simulink model "Example_IOBlock_Library_CAN"  (Simulink 10.3)
settings: Solver=FixedStepDiscrete  StartTime=0.0  StopTime=10.0  FixedStep=0.01  RelTol=1e-3
libraries: IOBlock_Library_TTC580 x18, simulink x2
settings Model: Creator=hokka  LastModifiedBy=knovakovic  MultithreadedSim=on
settings Model: SuppressorTable=|
  | <?xml version="1.0" encoding="UTF-8" standalone="yes" ?>
  | <!DOCTYPE boost_serialization>
  | <boost_serialization signature="serialization::archive" version="17">
  | <DiagnosticSuppressor class_id="0" tracking_level="0" version="7">
  | 	<Table class_id="1" tracking_level="0" version="0">
  | 		<count>4</count>
  | 		<bucket_count>8</bucket_count>
  | 		<item_version>0</item_version>
  | 		<item class_id="2" tracking_level="0" version="0">
  | 			<first class_id="3" tracking_level="0" version="7">
  | 				<Source class_id="4" tracking_level="0" version="0">
  | 					<count>1</count>
  | 					<item_version>0</item_version>
  | 					<item>57:2245</item>
  | 				</Source>
  | 			</first>
  | 			<second class_id="5" tracking_level="0" version="7">
  | 				<SuppressedData class_id="6" tracking_level="0" version="0">
  | 					<count>2</count>
  | 					<bucket_count>8</bucket_count>
  | 					<item_version>0</item_version>
  | 					<item class_id="7" tracking_level="0" version="0">
  | 						<first class_id="8" tracking_level="0" version="7">
  | 							<ID>SimulinkFixedPoint:util:Overflowoccurred</ID>
  | 							<Cause>
  | 								<Source>
  | 									<count>0</count>
  | 									<item_version>0</item_version>
  | 								</Source>
  | 							</Cause>
  | 						</first>
  | 						<second class_id="9" tracking_level="0" version="7">
  | 							<Comment></Comment>
  | 							<User></User>
  | 							<LastModified class_id="10" tracking_level="0" version="0">
  | 								<ptime_date class_id="11" tracking_level="0" version="0">
  | 									<date>20160608</date>
  | 								</ptime_date>
  | 								<ptime_time_duration class_id="12" tracking_level="0" version="1">
  | 									<is_special>0</is_special>
  | 									<time_duration_hours>15</time_duration_hours>
  | 									<time_duration_minutes>23</time_duration_minutes>
  | 									<time_duration_seconds>17</time_duration_seconds>
  | 									<time_duration_fractional_seconds>0</time_duration_fractional_seconds>
  | 								</ptime_time_duration>
  | 							</LastModified>
  | 							<SuppressionType>1</SuppressionType>
  | 						</second>
  | 					</item>
  | 					<item>
  | 						<first>
  | 							<ID>Simulink:DataType:WarningOverFlowDetected</ID>
  | 							<Cause>
  | 								<Source>
  | 									<count>0</count>
  | 									<item_version>0</item_version>
  | 								</Source>
  | 							</Cause>
  | 						</first>
  | 						<second>
  | 							<Comment></Comment>
  | 							<User></User>
  | 							<LastModified>
  | 								<ptime_date>
  | 									<date>20160608</date>
  | 								</ptime_date>
  | 								<ptime_time_duration>
  | 									<is_special>0</is_special>
  | 									<time_duration_hours>15</time_duration_hours>
  | 									<time_duration_minutes>23</time_duration_minutes>
  | 									<time_duration_seconds>17</time_duration_seconds>
  | 									<time_duration_fractional_seconds>0</time_duration_fractional_seconds>
  | 								</ptime_time_duration>
  | 							</LastModified>
  | 							<SuppressionType>1</SuppressionType>
  | 						</second>
  | 					</item>
  | 				</SuppressedData>
  | 			</second>
  | 		</item>
  | 		<item>
  | 			<first>
  | 				<Source>
  | 					<count>1</count>
  | 					<item_version>0</item_version>
  | 					<item>56:2245</item>
  | 				</Source>
  | 			</first>
  | 			<second>
  | 				<SuppressedData>
  | 					<count>2</count>
  | 					<bucket_count>8</bucket_count>
  | 					<item_version>0</item_version>
  | 					<item>
  | 						<first>
  | 							<ID>SimulinkFixedPoint:util:Overflowoccurred</ID>
  | 							<Cause>
  | 								<Source>
  | 									<count>0</count>
  | 									<item_version>0</item_version>
  | 								</Source>
  | 							</Cause>
  | 						</first>
  | 						<second>
  | 							<Comment></Comment>
  | 							<User></User>
  | 							<LastModified>
  | 								<ptime_date>
  | 									<date>20160608</date>
  | 								</ptime_date>
  | 								<ptime_time_duration>
  | 									<is_special>0</is_special>
  | 									<time_duration_hours>15</time_duration_hours>
  | 									<time_duration_minutes>23</time_duration_minutes>
  | 									<time_duration_seconds>17</time_duration_seconds>
  | 									<time_duration_fractional_seconds>0</time_duration_fractional_seconds>
  | 								</ptime_time_duration>
  | 							</LastModified>
  | 							<SuppressionType>1</SuppressionType>
  | 						</second>
  | 					</item>
  | 					<item>
  | 						<first>
  | 							<ID>Simulink:DataType:WarningOverFlowDetected</ID>
  | 							<Cause>
  | 								<Source>
  | 									<count>0</count>
  | 									<item_version>0</item_version>
  | 								</Source>
  | 							</Cause>
  | 						</first>
  | 						<second>
  | 							<Comment></Comment>
  | 							<User></User>
  | 							<LastModified>
  | 								<ptime_date>
  | 									<date>20160608</date>
  | 								</ptime_date>
  | 								<ptime_time_duration>
  | 									<is_special>0</is_special>
  | 									<time_duration_hours>15</time_duration_hours>
  | 									<time_duration_minutes>23</time_duration_minutes>
  | 									<time_duration_seconds>17</time_duration_seconds>
  | 									<time_duration_fractional_seconds>0</time_duration_fractional_seconds>
  | 								</ptime_time_duration>
  | 							</LastModified>
  | 							<SuppressionType>1</SuppressionType>
  | 						</second>
  | 					</item>
  | 				</SuppressedData>
  | 			</second>
  | 		</item>
  | 		<item>
  | 			<first>
  | 				<Source>
  | 					<count>1</count>
  | 					<item_version>0</item_version>
  | 					<item>58:2245</item>
  | 				</Source>
  | 			</first>
  | 			<second>
  | 				<SuppressedData>
  | 					<count>2</count>
  | 					<bucket_count>8</bucket_count>
  | 					<item_version>0</item_version>
  | 					<item>
  | 						<first>
  | 							<ID>SimulinkFixedPoint:util:Overflowoccurred</ID>
  | 							<Cause>
  | 								<Source>
  | 									<count>0</count>
  | 									<item_version>0</item_version>
  | 								</Source>
  | 							</Cause>
  | 						</first>
  | 						<second>
  | 							<Comment></Comment>
  | 							<User></User>
  | 							<LastModified>
  | 								<ptime_date>
  | 									<date>20160608</date>
  | 								</ptime_date>
  | 								<ptime_time_duration>
  | 									<is_special>0</is_special>
  | 									<time_duration_hours>15</time_duration_hours>
  | 									<time_duration_minutes>23</time_duration_minutes>
  | 									<time_duration_seconds>17</time_duration_seconds>
  | 									<time_duration_fractional_seconds>0</time_duration_fractional_seconds>
  | 								</ptime_time_duration>
  | 							</LastModified>
  | 							<SuppressionType>1</SuppressionType>
  | 						</second>
  | 					</item>
  | 					<item>
  | 						<first>
  | 							<ID>Simulink:DataType:WarningOverFlowDetected</ID>
  | 							<Cause>
  | 								<Source>
  | 									<count>0</count>
  | 									<item_version>0</item_version>
  | 								</Source>
  | 							</Cause>
  | 						</first>
  | 						<second>
  | 							<Comment></Comment>
  | 							<User></User>
  | 							<LastModified>
  | 								<ptime_date>
  | 									<date>20160608</date>
  | 								</ptime_date>
  | 								<ptime_time_duration>
  | 									<is_special>0</is_special>
  | 									<time_duration_hours>15</time_duration_hours>
  | 									<time_duration_minutes>23</time_duration_minutes>
  | 									<time_duration_seconds>17</time_duration_seconds>
  | 									<time_duration_fractional_seconds>0</time_duration_fractional_seconds>
  | 								</ptime_time_duration>
  | 							</LastModified>
  | 							<SuppressionType>1</SuppressionType>
  | 						</second>
  | 					</item>
  | 				</SuppressedData>
  | 			</second>
  | 		</item>
  | 		<item>
  | 			<first>
  | 				<Source>
  | 					<count>1</count>
  | 					<item_version>0</item_version>
  | 					<item>55:250</item>
  | 				</Source>
  | 			</first>
  | 			<second>
  | 				<SuppressedData>
  | 					<count>2</count>
  | 					<bucket_count>8</bucket_count>
  | 					<item_version>0</item_version>
  | 					<item>
  | 						<first>
  | 							<ID>SimulinkFixedPoint:util:Overflowoccurred</ID>
  | 							<Cause>
  | 								<Source>
  | 									<count>0</count>
  | 									<item_version>0</item_version>
  | 								</Source>
  | 							</Cause>
  | 						</first>
  | 						<second>
  | 							<Comment></Comment>
  | 							<User></User>
  | 							<LastModified>
  | 								<ptime_date>
  | 									<date>20160608</date>
  | 								</ptime_date>
  | 								<ptime_time_duration>
  | 									<is_special>0</is_special>
  | 									<time_duration_hours>15</time_duration_hours>
  | 									<time_duration_minutes>23</time_duration_minutes>
  | 									<time_duration_seconds>17</time_duration_seconds>
  | 									<time_duration_fractional_seconds>0</time_duration_fractional_seconds>
  | 								</ptime_time_duration>
  | 							</LastModified>
  | 							<SuppressionType>1</SuppressionType>
  | 						</second>
  | 					</item>
  | 					<item>
  | 						<first>
  | 							<ID>Simulink:DataType:WarningOverFlowDetected</ID>
  | 							<Cause>
  | 								<Source>
  | 									<count>0</count>
  | 									<item_version>0</item_version>
  | 								</Source>
  | 							</Cause>
  | 						</first>
  | 						<second>
  | 							<Comment></Comment>
  | 							<User></User>
  | 							<LastModified>
  | 								<ptime_date>
  | 									<date>20160608</date>
  | 								</ptime_date>
  | 								<ptime_time_duration>
  | 									<is_special>0</is_special>
  | 									<time_duration_hours>15</time_duration_hours>
  | 									<time_duration_minutes>23</time_duration_minutes>
  | 									<time_duration_seconds>17</time_duration_seconds>
  | 									<time_duration_fractional_seconds>0</time_duration_fractional_seconds>
  | 								</ptime_time_duration>
  | 							</LastModified>
  | 							<SuppressionType>1</SuppressionType>
  | 						</second>
  | 					</item>
  | 				</SuppressedData>
  | 			</second>
  | 		</item>
  | 	</Table>
  | </DiagnosticSuppressor>
  | 
  | </boost_serialization>
  | 
  | </boost_serialization>
settings DataIOCC: LimitDataPoints=on
settings OptimizationCC: InitFltsAndDblsToZero=on  LifeSpan=1  EfficientTunableParamExpr=on
settings DebuggingCC: SolverPrmCheckMsg=warning  InheritedTsInSrcMsg=none
settings HardwareCC: ProdLargestAtomicInteger=Long  ProdLargestAtomicFloat=Double  ProdIntDivRoundTo=Zero  ProdEndianess=BigEndian  ProdHWDeviceType=Texas Instruments->TMS570 Cortex-R4
settings SFSimCC: MATLABDynamicMemAlloc=off
settings RTWCC: Description=Real-Time Workshop Embedded Coder (no auto configuration)  SystemTargetFile=ert.tlc  GenCodeOnly=on  TemplateMakefile=ert_TTC580.tmf
settings CodeAppCC: IgnoreCustomStorageClasses=off  CustomSymbolStrType=$N$R$M  InternalIdentifier=Classic
settings ERTTargetCC: MultiwordLength=2048  SupportAbsoluteTime=off  SupportNonFinite=off  ERTCustomFileTemplate=example_file_process.tlc  ConvertIfToSwitch=off  SuppressUnreachableDefaultCases=off
settings ConfigComp: CovSFcnEnable=off

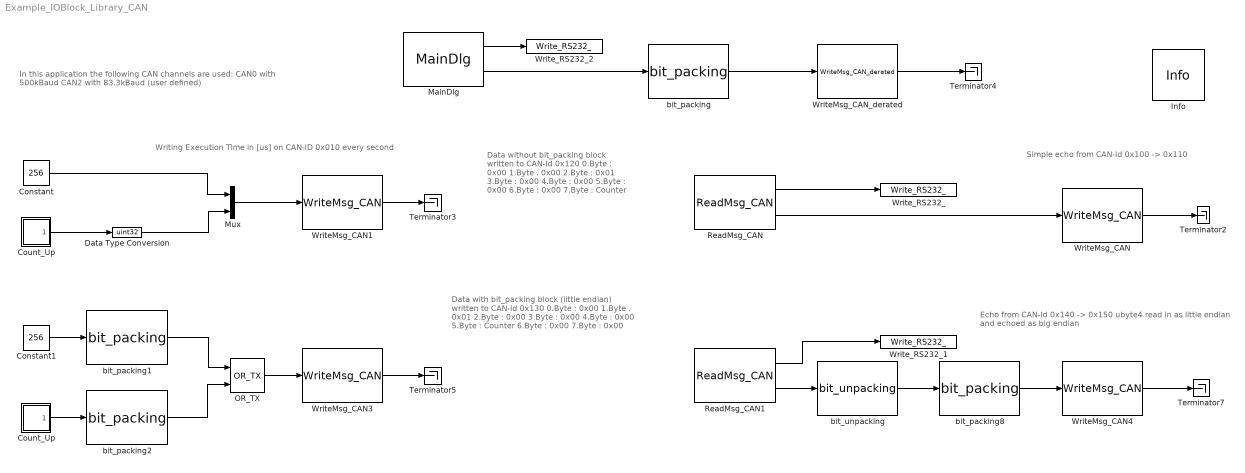
== system Example_IOBlock_Library_CAN ==
  note: Simple echo from CAN-Id 0x100 -> 0x110
  note: Data without bit_packing block
      | written to CAN-Id 0x120
      | 0.Byte : 0x00
      | 1.Byte . 0x00
      | 2.Byte : 0x01
      | 3.Byte : 0x00
      | 4.Byte : 0x00
      | 5.Byte : 0x00
      | 6.Byte : 0x00
      | 7.Byte : Counter
  note: Writing Execution Time in [us] on CAN-ID 0x010 every second
  note: Data with bit_packing block (little endian)
      | written to CAN-Id 0x130
      | 0.Byte : 0x00
      | 1.Byte . 0x01
      | 2.Byte : 0x00
      | 3.Byte : 0x00
      | 4.Byte : 0x00
      | 5.Byte : Counter
      | 6.Byte : 0x00
      | 7.Byte : 0x00
  note: Echo from CAN-Id 0x140 -> 0x150
      | ubyte4 read in as little endian and echoed as big endian
  note: In this application the following CAN channels are used:
      | CAN0 with 500kBaud
      | CAN2 with 83.3kBaud (user defined)
  Constant : Constant  Value=256  OutDataTypeStr=uint32
  Constant1 : Constant  Value=256  OutDataTypeStr=uint16
  Count_Up : Subsystem  mask{min_value=0, max_value=255, derate=100}
      mask prompts: derate "n-th step"
      mask help: Increment output every n-th step from min_value to max_value, then start from min_value again.
  "Count_Up " : Subsystem  mask{min_value=0, max_value=255, derate=100}
      mask prompts: derate "n-th step"
      mask help: Increment output every n-th step from min_value to max_value, then start from min_value again.
  Data Type Conversion : DataTypeConversion  OutDataTypeStr=uint32
  Info : IOBlock_Library_TTC580/Examples/Info  bla=0
      settings: SourceProductName=I/O Blocklibrary for TTC580
  MainDlg : IOBlock_Library_TTC580/System  Blocks TTC580 IOlib/MainDlg  Priority=-2147483646  SampleTime=-1  ttlib=IO_Blk_Lib_TTC500  ttDescription=MainDlg  tt_iolib_version=0.25  baudrate_CAN0=500  tseg1_CAN0=6  tseg2_CAN0=2  sjw_CAN0=1  brp_CAN0=1  baudrate_CAN1=500  tseg1_CAN1=6  tseg2_CAN1=2  sjw_CAN1=1  brp_CAN1=1  baudrate_CAN2=IO_CAN_BIT_USER  tseg1_CAN2=8  tseg2_CAN2=3  sjw_CAN2=1  brp_CAN2=8  baudrate_CAN3=500  baudrate_CAN4=500  baudrate_CAN5=500  baudrate_CAN6=500  tseg1=6  tseg2=2  sjw=1  Duration_ms=10  glitch_filter_time=180  watchdog_window_size=SAFETY_CONF_WINDOW_SIZE_100_PERCENT  watchdog_reset_behavior=SAFETY_CONF_RESETS_DISABLED  brp=0  Enable_sending_DM1_of_J1939=off  DM1_Channel=IO_CAN_CHANNEL_0  J1939SorceAddress=0  DM2_Basis_Address=63488  Show_version_information=off  Major_Number=0  Minor_Number=1  Revison_Number=1  Node_Number=1  Enable_Reset_by_TTCDownloader=on  bFlashOverEthernet=off  Enable_CCP=off  CRO_ID=hex2dec('101')  DTO_ID=hex2dec('102')  CCP_Station_Addr_raw=1  CCP_Station_ID=ECU00001  CPP_channel=IO_CAN_CHANNEL_0  CPP_id_format=IO_CAN_STD_FRAME  bEnable_DAQ0=off  bEnable_DAQ1_2=off  ODT_total=10  bEnable_ErrorCBAction=off  bDIAG_ERR_DISABLE_SSW0=off  bDIAG_ERR_DISABLE_SSW1=off  bDIAG_ERR_DISABLE_SSW2=off
      settings: SourceProductName=I/O Blocklibrary for TTC580
  Mux : Mux  Inputs=2
  OR_TX : IOBlock_Library_TTC580/CAN  Blocks TTC580 IOlib/OR_TX  logicop=OR  UseBitMask=off  NumInputPorts=2  BitMask=bin2dec('11011001')  BitMaskRealWorld=Stored Integer
      settings: SourceProductName=I/O Blocklibrary for TTC580
  ReadMsg_CAN : IOBlock_Library_TTC580/CAN  Blocks TTC580 IOlib/ReadMsg_CAN  SampleTime=-1  ttlib=IO_Blk_Lib_TTC500  ttDescription=ReadMsg_CAN  tt_iolib_version=0.26  channel=IO_CAN_CHANNEL_0  mode=IO_CAN_MSG_READ  id_format=IO_CAN_STD_FRAME  id=hex2dec('100')
      settings: SourceProductName=I/O Blocklibrary for TTC580
  ReadMsg_CAN1 : IOBlock_Library_TTC580/CAN  Blocks TTC580 IOlib/ReadMsg_CAN  SampleTime=-1  ttlib=IO_Blk_Lib_TTC500  ttDescription=ReadMsg_CAN  tt_iolib_version=0.26  channel=IO_CAN_CHANNEL_0  mode=IO_CAN_MSG_READ  id_format=IO_CAN_STD_FRAME  id=hex2dec('140')
      settings: SourceProductName=I/O Blocklibrary for TTC580
  Terminator{2..5,7} (5 alike) : Terminator
  WriteMsg_CAN : IOBlock_Library_TTC580/CAN  Blocks TTC580 IOlib/WriteMsg_CAN  SampleTime=-1  ttlib=IO_Blk_Lib_TTC500  ttDescription=WriteMsg_CAN  tt_iolib_version=0.26  channel=IO_CAN_CHANNEL_0  mode=IO_CAN_MSG_WRITE  id_format=IO_CAN_STD_FRAME  id=hex2dec('110')  length=8
      settings: SourceProductName=I/O Blocklibrary for TTC580
  WriteMsg_CAN1 : IOBlock_Library_TTC580/CAN  Blocks TTC580 IOlib/WriteMsg_CAN  SampleTime=-1  ttlib=IO_Blk_Lib_TTC500  ttDescription=WriteMsg_CAN  tt_iolib_version=0.26  channel=IO_CAN_CHANNEL_0  mode=IO_CAN_MSG_WRITE  id_format=IO_CAN_STD_FRAME  id=hex2dec('120')  length=8
      settings: SourceProductName=I/O Blocklibrary for TTC580
  WriteMsg_CAN3 : IOBlock_Library_TTC580/CAN  Blocks TTC580 IOlib/WriteMsg_CAN  SampleTime=-1  ttlib=IO_Blk_Lib_TTC500  ttDescription=WriteMsg_CAN  tt_iolib_version=0.26  channel=IO_CAN_CHANNEL_0  mode=IO_CAN_MSG_WRITE  id_format=IO_CAN_STD_FRAME  id=hex2dec('130')  length=8
      settings: SourceProductName=I/O Blocklibrary for TTC580
  WriteMsg_CAN4 : IOBlock_Library_TTC580/CAN  Blocks TTC580 IOlib/WriteMsg_CAN  SampleTime=-1  ttlib=IO_Blk_Lib_TTC500  ttDescription=WriteMsg_CAN  tt_iolib_version=0.26  channel=IO_CAN_CHANNEL_0  mode=IO_CAN_MSG_WRITE  id_format=IO_CAN_STD_FRAME  id=hex2dec('150')  length=8
      settings: SourceProductName=I/O Blocklibrary for TTC580
  WriteMsg_CAN_derated : IOBlock_Library_TTC580/CAN  Blocks TTC580 IOlib/WriteMsg_CAN_derated  SampleTime=-1  ttlib=IO_Blk_Lib_TTC500  ttDescription=WriteMsg_CAN_derated  tt_iolib_version=0.26  channel=IO_CAN_CHANNEL_2  mode=IO_CAN_MSG_WRITE  id_format=IO_CAN_STD_FRAME  id=hex2dec('10')  length=8  derate=100
      settings: SourceProductName=I/O Blocklibrary for TTC580
  Write_RS232_ : IOBlock_Library_TTC580/UART TTC580 IOlib/Write_RS232_  Priority=10  SampleTime=-1  ttlib=IO_Blk_Lib_TTC500  ttDescription=Write_RS232_  tt_iolib_version=0.25  Comment=ReadCANId 0x100 ErrorCode =
      settings: SourceProductName=I/O Blocklibrary for TTC580
  Write_RS232_1 : IOBlock_Library_TTC580/UART TTC580 IOlib/Write_RS232_  Priority=20  SampleTime=-1  ttlib=IO_Blk_Lib_TTC500  ttDescription=Write_RS232_  tt_iolib_version=0.25  Comment=ReadCANId 0x140 ErrorCode =
      settings: SourceProductName=I/O Blocklibrary for TTC580
  Write_RS232_2 : IOBlock_Library_TTC580/UART TTC580 IOlib/Write_RS232_  Priority=0  SampleTime=-1  ttlib=IO_Blk_Lib_TTC500  ttDescription=Write_RS232_  tt_iolib_version=0.25  Comment=ErrorCode MainDlg =
      settings: SourceProductName=I/O Blocklibrary for TTC580
  bit_packing : IOBlock_Library_TTC580/CAN  Blocks TTC580 IOlib/bit_packing  SampleTime=-1  ttlib=IO_Blk_Lib_TTC500  ttDescription=bit_packing  tt_iolib_version=0.26  Endianness=little  Format=unsigned  Inversion=off  Startbit=0  Width_bits=32  Factor=1.0  Offset=0.0
      settings: SourceProductName=I/O Blocklibrary for TTC580
  bit_packing1 : IOBlock_Library_TTC580/CAN  Blocks TTC580 IOlib/bit_packing  SampleTime=-1  ttlib=IO_Blk_Lib_TTC500  ttDescription=bit_packing  tt_iolib_version=0.26  Endianness=little  Format=unsigned  Inversion=off  Startbit=0  Width_bits=16  Factor=1.0  Offset=0.0
      settings: SourceProductName=I/O Blocklibrary for TTC580
  bit_packing2 : IOBlock_Library_TTC580/CAN  Blocks TTC580 IOlib/bit_packing  SampleTime=-1  ttlib=IO_Blk_Lib_TTC500  ttDescription=bit_packing  tt_iolib_version=0.26  Endianness=little  Format=unsigned  Inversion=off  Startbit=40  Width_bits=8  Factor=1.0  Offset=0.0
      settings: SourceProductName=I/O Blocklibrary for TTC580
  bit_packing8 : IOBlock_Library_TTC580/CAN  Blocks TTC580 IOlib/bit_packing  SampleTime=-1  ttlib=IO_Blk_Lib_TTC500  ttDescription=bit_packing  tt_iolib_version=0.26  Endianness=big  Format=unsigned  Inversion=off  Startbit=24  Width_bits=32  Factor=1.0  Offset=0.0
      settings: SourceProductName=I/O Blocklibrary for TTC580
  bit_unpacking : IOBlock_Library_TTC580/CAN  Blocks TTC580 IOlib/bit_unpacking  SampleTime=-1  ttlib=IO_Blk_Lib_TTC500  ttDescription=bit_unpacking  tt_iolib_version=0.26  Endianness=little  Format=unsigned  Inversion=off  Startbit=0  Width_bits=32  Factor=1.0  Offset=0.0
      settings: SourceProductName=I/O Blocklibrary for TTC580
  wires:
  ReadMsg_CAN/1 -> Write_RS232_/1
  ReadMsg_CAN/2 -> WriteMsg_CAN/1
  WriteMsg_CAN/1 -> Terminator2/1
  WriteMsg_CAN1/1 -> Terminator3/1
  Constant/1 -> Mux/1
  Mux/1 -> WriteMsg_CAN1/1
  Count_Up/1(Out1) -> Data Type Conversion/1
  Data Type Conversion/1 -> Mux/2
  WriteMsg_CAN_derated/1 -> Terminator4/1
  bit_packing/1 -> WriteMsg_CAN_derated/1
  WriteMsg_CAN3/1 -> Terminator5/1
  "Count_Up "/1(Out1) -> bit_packing2/1
  Constant1/1 -> bit_packing1/1
  bit_packing1/1 -> OR_TX/1
  bit_packing2/1 -> OR_TX/2
  OR_TX/1 -> WriteMsg_CAN3/1
  ReadMsg_CAN1/1 -> Write_RS232_1/1
  WriteMsg_CAN4/1 -> Terminator7/1
  bit_packing8/1 -> WriteMsg_CAN4/1
  ReadMsg_CAN1/2 -> bit_unpacking/1
  bit_unpacking/1 -> bit_packing8/1
  MainDlg/2 -> bit_packing/1
  MainDlg/1 -> Write_RS232_2/1

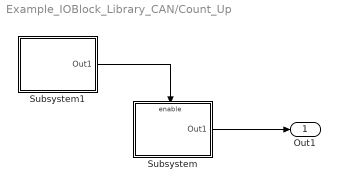
== system Example_IOBlock_Library_CAN/Count_Up ==
  Subsystem : Subsystem  mask{min_value=min_value, max_value=max_value}
      mask help: Increment output from min to max_value, then start from min again.
  Subsystem1 : Subsystem  mask{max_value=derate}
      mask help: Increment output from 0 to max_value, then start from 0 again.
  Out1 : Outport  VectorParamsAs1DForOutWhenUnconnected=off
  wires:
  Subsystem/1(Out1) -> Out1/1
  Subsystem1/1(Out1) -> Subsystem/Enable

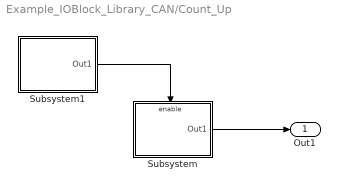
== system Example_IOBlock_Library_CAN/Count_Up  ==
  Subsystem : Subsystem  mask{min_value=min_value, max_value=max_value}
      mask help: Increment output from min to max_value, then start from min again.
  Subsystem1 : Subsystem  mask{max_value=derate}
      mask help: Increment output from 0 to max_value, then start from 0 again.
  Out1 : Outport  VectorParamsAs1DForOutWhenUnconnected=off
  wires:
  Subsystem1/1(Out1) -> Subsystem/Enable
  Subsystem/1(Out1) -> Out1/1

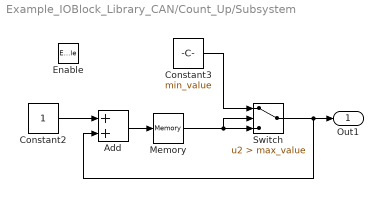
== system Example_IOBlock_Library_CAN/Count_Up/Subsystem ==
  Enable : EnablePort
  Add : Sum
  Constant2 : Constant  OutDataTypeStr=uint16
  Constant3 : Constant  Value=min_value  OutDataTypeStr=uint16
  Memory : Memory  InitialCondition=min_value
  Switch : Switch  Criteria=u2 > Threshold  Threshold=max_value  OutDataTypeStr=uint16
  Out1 : Outport  VectorParamsAs1DForOutWhenUnconnected=off
  wires:
  Constant2/1 -> Add/1
  Add/1 -> Memory/1
  Memory/1 -> Switch/3, Switch/2
  Switch/1 -> Out1/1, Add/2
  Constant3/1 -> Switch/1

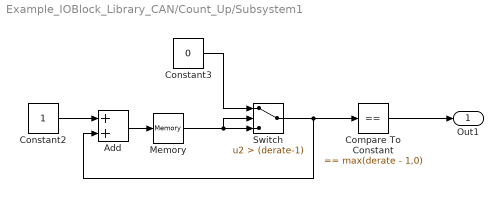
== system Example_IOBlock_Library_CAN/Count_Up/Subsystem1 ==
  Add : Sum
  Compare To Constant : simulink/Logic and Bit Operations/Compare To Constant  relop===  const=max(derate - 1,0)  OutDataTypeStr=boolean  ZeroCross=off
  Constant2 : Constant  OutDataTypeStr=uint16
  Constant3 : Constant  Value=0  OutDataTypeStr=uint16
  Memory : Memory
  Switch : Switch  Criteria=u2 > Threshold  Threshold=(derate-1)  OutDataTypeStr=uint16
  Out1 : Outport  VectorParamsAs1DForOutWhenUnconnected=off
  wires:
  Constant3/1 -> Switch/1
  Switch/1 -> Add/2, Compare To Constant/1
  Memory/1 -> Switch/2, Switch/3
  Add/1 -> Memory/1
  Constant2/1 -> Add/1
  Compare To Constant/1 -> Out1/1

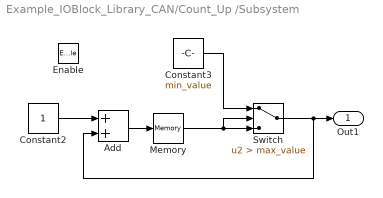
== system Example_IOBlock_Library_CAN/Count_Up /Subsystem ==
  Enable : EnablePort
  Add : Sum
  Constant2 : Constant  OutDataTypeStr=uint16
  Constant3 : Constant  Value=min_value  OutDataTypeStr=uint16
  Memory : Memory  InitialCondition=min_value
  Switch : Switch  Criteria=u2 > Threshold  Threshold=max_value  OutDataTypeStr=uint16
  Out1 : Outport  VectorParamsAs1DForOutWhenUnconnected=off
  wires:
  Constant3/1 -> Switch/1
  Switch/1 -> Add/2, Out1/1
  Memory/1 -> Switch/2, Switch/3
  Add/1 -> Memory/1
  Constant2/1 -> Add/1

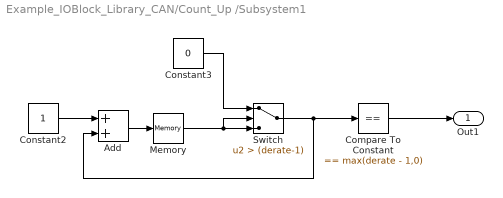
== system Example_IOBlock_Library_CAN/Count_Up /Subsystem1 ==
  Add : Sum
  Compare To Constant : simulink/Logic and Bit Operations/Compare To Constant  relop===  const=max(derate - 1,0)  OutDataTypeStr=boolean  ZeroCross=off
  Constant2 : Constant  OutDataTypeStr=uint16
  Constant3 : Constant  Value=0  OutDataTypeStr=uint16
  Memory : Memory
  Switch : Switch  Criteria=u2 > Threshold  Threshold=(derate-1)  OutDataTypeStr=uint16
  Out1 : Outport  VectorParamsAs1DForOutWhenUnconnected=off
  wires:
  Compare To Constant/1 -> Out1/1
  Constant2/1 -> Add/1
  Add/1 -> Memory/1
  Memory/1 -> Switch/3, Switch/2
  Switch/1 -> Compare To Constant/1, Add/2
  Constant3/1 -> Switch/1
